simulink model "simulated_pins"  (R2021a)
settings: Solver=VariableStepAuto  StartTime=0.0  StopTime=3  RelTol=1e-3
values from neighbouring files (symbols this model uses):
  A = zeros(5,5)    [ATV_5.m]    (also in ATV_LAB_MODELAGEM_TERMODINAMICA.m; ATV_LAB_MODELAGEM_TERMODINAMICA_simulink.m)
  B = zeros(5,2)    [ATV_5.m]    (also in ATV_LAB_MODELAGEM_TERMODINAMICA.m = zeros(5,5); ATV_LAB_MODELAGEM_TERMODINAMICA_simulink.m)
  C = eye(5)    [ATV_5.m]    (also in ATV_LAB_MODELAGEM_TERMODINAMICA.m; ATV_LAB_MODELAGEM_TERMODINAMICA_simulink.m)
  D = zeros(5,2)    [ATV_5.m]    (also in ATV_LAB_MODELAGEM_TERMODINAMICA.m = zeros(5,5); ATV_LAB_MODELAGEM_TERMODINAMICA_simulink.m)
settings Model: Creator=Home  LastModifiedBy=Home

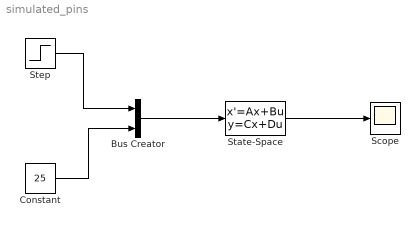
== system simulated_pins ==
  Bus Creator : BusCreator  Inputs=2
  Constant : Constant  Value=25
  Scope : Scope
  State-Space : StateSpace  A=A  B=B  C=C  D=D  InitialCondition=0
  Step : Step  Time=0  After=100  SampleTime=0
  wires:
  Bus Creator/1 -> State-Space/1
  Constant/1 -> Bus Creator/2
  Step/1 -> Bus Creator/1
  State-Space/1 -> Scope/1
